simulink model "ITSC2021_CoupledPathFollowingSim_discrete"  (R2019b)
settings: Solver=FixedStepAuto  StartTime=0.0  StopTime=50  FixedStep=0.01  RelTol=1e-4  EnableMultiTasking=on
values from neighbouring files (symbols this model uses):
  friction_grid_cluster = [frictionGrid_Cluster_table.position_x, frictionGrid_Cluster_table.position_y, frictionGrid_Cluster_table.position_z, frictionGrid_Cluster_table.friction_coefficient]    [ITSC2021_runCoupledPathFollowingSim.m]
  inputTrajectory = inputTrajectory(unique_station_indices,:)    [ITSC2021_runCoupledPathFollowingSim.m]
  road_geometry = [sectionRef_table.east, sectionRef_table.north, sectionRef_table.up, sectionRef_table.grade, sectionRef_table.bank, road_geometry_radius, sectionRef_table.yaw]    [ITSC2021_runCoupledPathFollowingSim.m]
undefined symbols (not defined in the file or in its folder): DiscIntNeverNeededParam, flag, initial, mdlparam, mdlParam
libraries: simulink x6, autolibshared x1
(part 2 of 3)

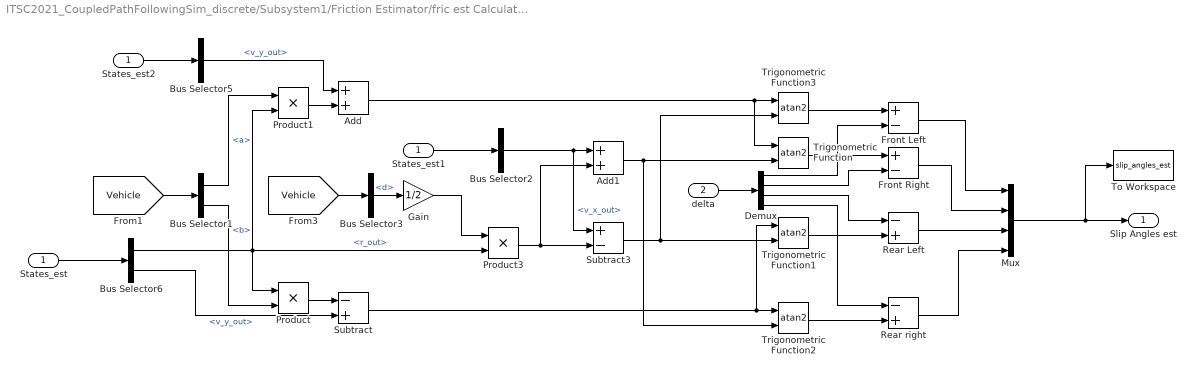
== system ITSC2021_CoupledPathFollowingSim_discrete/Subsystem1/Friction Estimator/fric est Calculate Slips ==
  States_est : Inport
  delta : Inport  Port=2
  Add : Sum
  Add1 : Sum
  Bus Selector1 : BusSelector  OutputSignals=a,b
  Bus Selector2 : BusSelector  OutputSignals=v_x_out
  Bus Selector3 : BusSelector  OutputSignals=d
  Bus Selector5 : BusSelector  OutputSignals=v_y_out
  Bus Selector6 : BusSelector  OutputSignals=r_out,v_y_out
  Demux : Demux
  Front Left : Sum  Inputs=+-
  Front Right : Sum  Inputs=+-
  Gain : Gain  Gain=1/2
  Mux : Mux
  Product : Product  RndMeth=Zero
  Product1 : Product  RndMeth=Zero
  Product3 : Product  RndMeth=Zero
  Rear Left : Sum  Inputs=-+
  Rear right : Sum  Inputs=-+
  States_est1 : InportShadow
  States_est2 : InportShadow
  Subtract : Sum  Inputs=-+
  Subtract3 : Sum  Inputs=+-
  To Workspace : ToWorkspace  VariableName=slip_angles_est  SampleTime=-1
  Trigonometric Function{,1..3} (4 alike) : Trigonometry  Operator=atan2
  Slip Angles est : Outport
  wires:
  Product1/1 -> Add/2
  Trigonometric Function3/1 -> Front Left/1
  Bus Selector1/1 -> Product1/1  "<a>"
  [Vehicle] -> Bus Selector3/1
  Front Left/1 -> Mux/1
  Front Right/1 -> Mux/2
  Bus Selector1/2 -> Product/2  "<b>"
  Trigonometric Function2/1 -> Rear right/2
  Mux/1 -> Slip Angles est/1, To Workspace/1
  Product/1 -> Subtract/1
  [Vehicle] -> Bus Selector1/1
  Add/1 -> Trigonometric Function3/1, Trigonometric Function/1
  Demux/3 -> Rear Left/1
  Demux/4 -> Rear right/1
  Bus Selector3/1 -> Gain/1  "<d>"
  Rear right/1 -> Mux/4
  Rear Left/1 -> Mux/3
  delta/1 -> Demux/1
  Gain/1 -> Product3/1
  Trigonometric Function/1 -> Front Right/1
  Subtract3/1 -> Trigonometric Function1/2, Trigonometric Function3/2
  Trigonometric Function1/1 -> Rear Left/2
  States_est/1 -> Bus Selector6/1
  Demux/2 -> Front Right/2
  Bus Selector6/2 -> Subtract/2  "<v_y_out>"
  Product3/1 -> Subtract3/2, Add1/2
  Add1/1 -> Trigonometric Function/2, Trigonometric Function2/2
  Subtract/1 -> Trigonometric Function2/1, Trigonometric Function1/1
  Demux/1 -> Front Left/2
  Bus Selector6/1 -> Product/1, Product1/2, Product3/2  "<r_out>"
  Bus Selector2/1 -> Subtract3/1, Add1/1  "<v_x_out>"
  States_est1/1 -> Bus Selector2/1
  States_est2/1 -> Bus Selector5/1
  Bus Selector5/1 -> Add/1  "<v_y_out>"

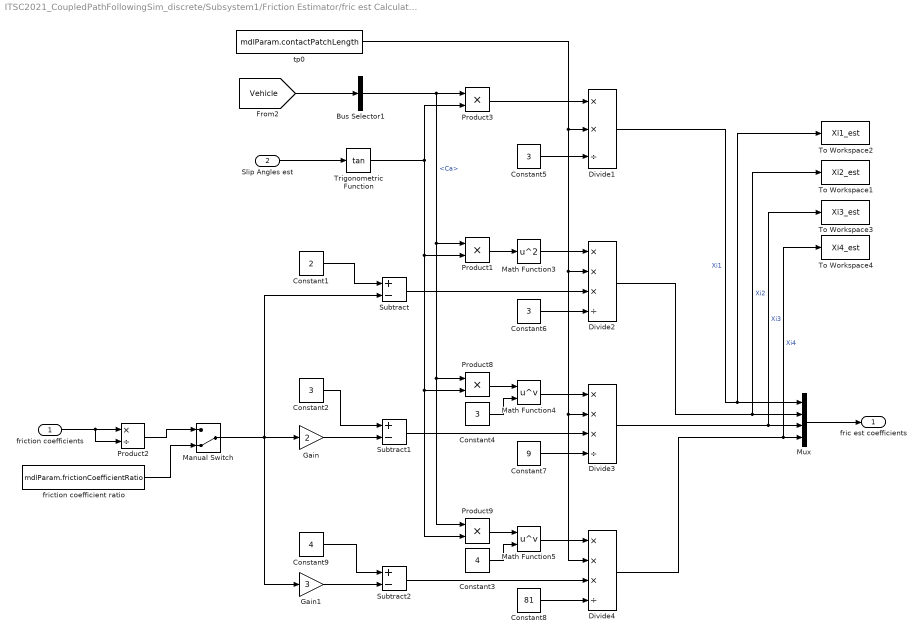
== system ITSC2021_CoupledPathFollowingSim_discrete/Subsystem1/Friction Estimator/fric est Calculate Xis ==
  friction coefficients : Inport
  Slip Angles est : Inport  Port=2
  Bus Selector1 : BusSelector  OutputSignals=Ca
  Constant1 : Constant  Value=2
  Constant{2,4..6} (4 alike) : Constant  Value=3
  Constant3 : Constant  Value=4
  Constant7 : Constant  Value=9
  Constant8 : Constant  Value=81
  Constant9 : Constant  Value=4
  Divide1 : Product  Inputs=**/
  Divide2 : Product  Inputs=***/
  Divide3 : Product  Inputs=***/
  Divide4 : Product  Inputs=***/
  Gain : Gain  Gain=2
  Gain1 : Gain  Gain=3
  Manual Switch : ManualSwitch  CurrentSetting=0
  Math Function3 : Math  Operator=square  SaturateOnIntegerOverflow=on
  Math Function4 : Math  Operator=pow  SignedPower=off  SaturateOnIntegerOverflow=on
  Math Function5 : Math  Operator=pow  SignedPower=off  SaturateOnIntegerOverflow=on
  Mux : Mux
  Product{1,3,8..9} (4 alike) : Product  RndMeth=Zero
  Product2 : Product  Inputs=*/  RndMeth=Zero
  Subtract : Sum  Inputs=+-
  Subtract1 : Sum  Inputs=+-
  Subtract2 : Sum  Inputs=+-
  To Workspace1 : ToWorkspace  VariableName=Xi2_est  SampleTime=-1
  To Workspace2 : ToWorkspace  VariableName=Xi1_est  SampleTime=-1
  To Workspace3 : ToWorkspace  VariableName=Xi3_est  SampleTime=-1
  To Workspace4 : ToWorkspace  VariableName=Xi4_est  SampleTime=-1
  Trigonometric Function : Trigonometry  Operator=tan
  friction coefficient ratio : Constant  Value=mdlParam.frictionCoefficientRatio
  tp0 : Constant  Value=mdlParam.contactPatchLength
  fric est coefficients : Outport
  wires:
  Mux/1 -> fric est coefficients/1
  Trigonometric Function/1 -> Product1/2, Product8/2, Product9/2, Product3/2
  tp0/1 -> Divide4/2, Divide3/2, Divide2/2, Divide1/2
  Bus Selector1/1 -> Product9/1, Product8/1, Product1/1, Product3/1  "<Ca>"
  Constant3/1 -> Math Function5/2
  Constant4/1 -> Math Function4/2
  Math Function3/1 -> Divide2/1
  Product1/1 -> Math Function3/1
  [Vehicle] -> Bus Selector1/1
  Math Function4/1 -> Divide3/1
  Constant5/1 -> Divide1/3
  Slip Angles est/1 -> Trigonometric Function/1
  Math Function5/1 -> Divide4/1
  Product8/1 -> Math Function4/1
  Product9/1 -> Math Function5/1
  Constant7/1 -> Divide3/4
  Product3/1 -> Divide1/1
  Subtract1/1 -> Divide3/3
  Constant1/1 -> Subtract/1
  Constant2/1 -> Subtract1/1
  Manual Switch/1 -> Gain1/1, Subtract/2, Gain/1
  Gain/1 -> Subtract1/2
  Constant9/1 -> Subtract2/1
  Gain1/1 -> Subtract2/2
  Constant6/1 -> Divide2/4
  Subtract/1 -> Divide2/3
  Constant8/1 -> Divide4/4
  Subtract2/1 -> Divide4/3
  Divide1/1 -> To Workspace2/1, Mux/1  "Xi1"
  Divide4/1 -> To Workspace4/1, Mux/4  "Xi4"
  Divide2/1 -> To Workspace1/1, Mux/2  "Xi2"
  Divide3/1 -> To Workspace3/1, Mux/3  "Xi3"
  friction coefficients/1 -> Product2/2, Product2/1
  Product2/1 -> Manual Switch/1
  friction coefficient ratio/1 -> Manual Switch/2

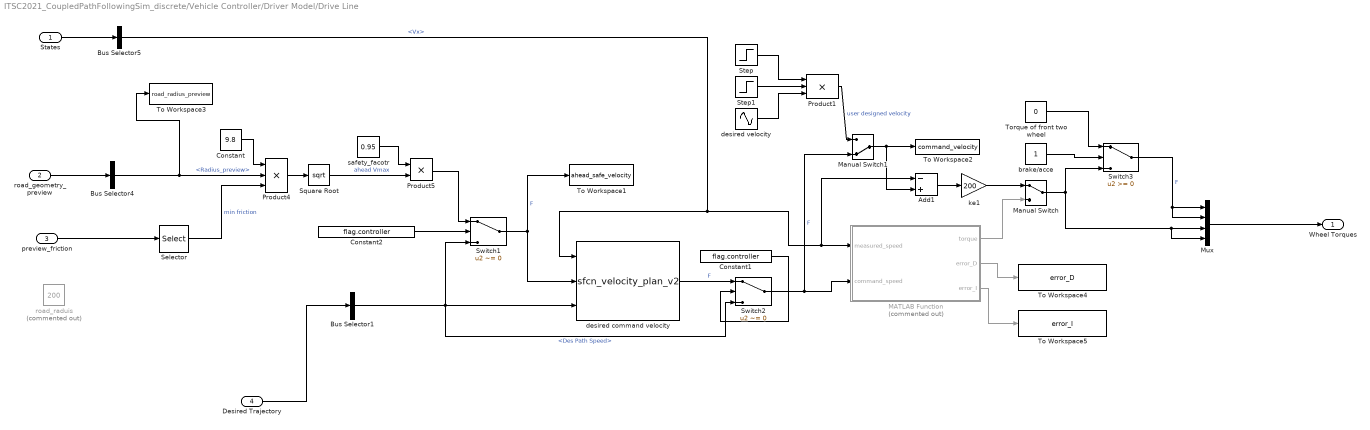
== system ITSC2021_CoupledPathFollowingSim_discrete/Vehicle Controller/Driver Model/Drive Line ==
  States : Inport
  road_geometry_preview : Inport  Port=2
  preview_friction : Inport  Port=3
  Desired Trajectory : Inport  Port=4
  Add1 : Sum  Inputs=-+
  Bus Selector1 : BusSelector  OutputSignals=Des Path Speed
  Bus Selector4 : BusSelector  OutputSignals=Radius_preview
  Bus Selector5 : BusSelector  OutputSignals=Vx
  Constant : Constant  Value=9.8
  Constant1 : Constant  Value=flag.controller
  Constant2 : Constant  Value=flag.controller
  MATLAB Function : MATLAB Function  Commented=on  TreatAsAtomicUnit=on
  Manual Switch : ManualSwitch
      settings: AttributesFormatString=%<BlockType>
  Manual Switch1 : ManualSwitch  CurrentSetting=0
  Mux : Mux
  Product1 : Product  Inputs=3  SaturateOnIntegerOverflow=on  OutDataTypeStr=Inherit: Same as first input
  Product4 : Product  Inputs=3
  Product5 : Product
  Selector : Selector  InputPortWidth=5  IndexOptions=Index vector (dialog)  Indices=[3]  OutputSizes=1
  Square Root : Sqrt  SaturateOnIntegerOverflow=on
  Step : Step  Time=2  Before=1  After=0.8  SampleTime=0.01
  Step1 : Step  Time=20  Before=1  After=1.2  SampleTime=0.01
  Switch1 : Switch  Criteria=u2 ~= 0  ZeroCross=off
  Switch2 : Switch  Criteria=u2 ~= 0  ZeroCross=off
  Switch3 : Switch  ZeroCross=off
  To Workspace1 : ToWorkspace  VariableName=ahead_safe_velocity  SampleTime=-1
      settings: Save2DSignal=2-D array (concatenate along first dimension)
  To Workspace2 : ToWorkspace  VariableName=command_velocity  SampleTime=-1
      settings: Save2DSignal=2-D array (concatenate along first dimension)
  To Workspace3 : ToWorkspace  VariableName=road_radius_preview  SampleTime=-1
      settings: Save2DSignal=2-D array (concatenate along first dimension)
  To Workspace4 : ToWorkspace  VariableName=error_D  SampleTime=-1
      settings: Save2DSignal=2-D array (concatenate along first dimension)
  To Workspace5 : ToWorkspace  VariableName=error_I  SampleTime=-1
      settings: Save2DSignal=2-D array (concatenate along first dimension)
  Torque of front two wheel : Constant  Value=0
  brake/acce : Constant
  desired command velocity : M-S-Function  FunctionName=sfcn_velocity_plan_v2
  desired velocity : Sin  SineType=Sample based  Amplitude=0  Bias=27.392001251200000  Frequency=0.1*2*pi  Samples=2000  SampleTime=0.01
  ke1 : Gain  Gain=200
  road_raduis : Constant  Commented=on  Value=200
  safety_facotr : Constant  Value=0.95
  Wheel Torques : Outport
  wires:
  Product4/1 -> Square Root/1
  Add1/1 -> ke1/1
  States/1 -> Bus Selector5/1
  Switch2/1 -> Manual Switch1/2, MATLAB Function/2(command_speed)  "F"
  Bus Selector5/1 -> Add1/1, MATLAB Function/1(measured_speed), desired command velocity/1  "<Vx>"
  Switch3/1 -> Mux/2, Mux/1  "F"
  Bus Selector1/1 -> Switch1/3, Switch2/3, desired command velocity/3  "<Des Path Speed>"
  Torque of front two wheel/1 -> Switch3/1
  Product5/1 -> Switch1/1
  Selector/1 -> Product4/3  "min friction"
  MATLAB Function/3(error_I) -> To Workspace5/1
  MATLAB Function/2(error_D) -> To Workspace4/1
  Manual Switch/1 -> Mux/4, Mux/3, Switch3/3
  Bus Selector4/1 -> To Workspace3/1, Product4/2  "<Radius_preview>"
  desired command velocity/1 -> Switch2/1  "F"
  Constant/1 -> Product4/1
  Constant2/1 -> Switch1/2
  Square Root/1 -> Product5/2  "ahead Vmax"
  brake/acce/1 -> Switch3/2
  Desired Trajectory/1 -> Bus Selector1/1
  Switch1/1 -> desired command velocity/2, To Workspace1/1  "F"
  ke1/1 -> Manual Switch/1
  safety_facotr/1 -> Product5/1
  MATLAB Function/1(torque) -> Manual Switch/2
  Constant1/1 -> Switch2/2
  road_geometry_preview/1 -> Bus Selector4/1
  preview_friction/1 -> Selector/1
  Mux/1 -> Wheel Torques/1
  desired velocity/1 -> Product1/3
  Step/1 -> Product1/1
  Product1/1 -> Manual Switch1/1  "user designed velocity"
  Step1/1 -> Product1/2
  Manual Switch1/1 -> To Workspace2/1, Add1/2

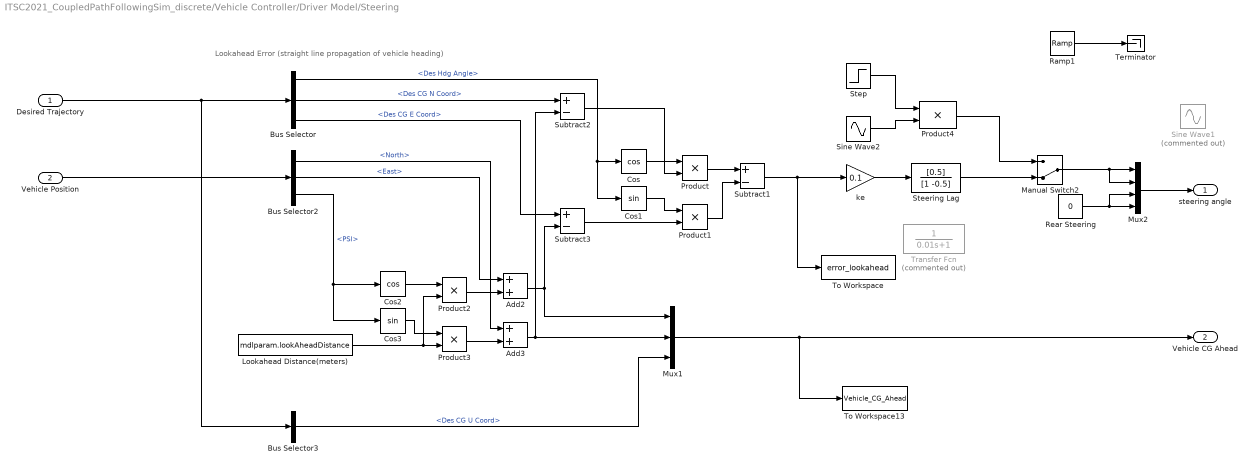
== system ITSC2021_CoupledPathFollowingSim_discrete/Vehicle Controller/Driver Model/Steering ==
  note: Lookahead Error (straight line propagation of vehicle heading)
  Desired Trajectory : Inport
  Vehicle Position : Inport  Port=2
  Add2 : Sum
  Add3 : Sum
  Bus Selector : BusSelector  OutputSignals=Des Hdg Angle,Des CG N Coord,Des CG E Coord
  Bus Selector2 : BusSelector  OutputSignals=North,East,PSI
  Bus Selector3 : BusSelector  OutputSignals=Des CG U Coord
  Cos : Trigonometry  Operator=cos
  Cos1 : Trigonometry
  Cos2 : Trigonometry  Operator=cos
  Cos3 : Trigonometry
  Lookahead Distance(meters) : Constant  Value=mdlparam.lookAheadDistance
  Manual Switch2 : ManualSwitch  CurrentSetting=0
  Mux1 : Mux  Inputs=3
  Mux2 : Mux
  Product{,1..3} (4 alike) : Product
  Product4 : Product  SaturateOnIntegerOverflow=on  OutDataTypeStr=Inherit: Same as first input
  Ramp1 : simulink/Sources/Ramp  slope=0.1  start=0  InitialOutput=0
  Rear Steering : Constant  Value=0
  Sine Wave1 : Sin  Commented=on  SampleTime=0
  Sine Wave2 : Sin  SineType=Sample based  Amplitude=0*pi/180  Frequency=0.1*2*pi  Samples=2000  SampleTime=0.01
  Steering Lag : DiscreteFilter  Numerator=[0.5]  Denominator=[1 -0.5]
  Step : Step  Time=40  Before=1  After=0  SampleTime=0.01
  Subtract1 : Sum  Inputs=+-
  Subtract2 : Sum  Inputs=+-
  Subtract3 : Sum  Inputs=+-
  Terminator : Terminator
  To Workspace : ToWorkspace  VariableName=error_lookahead  SampleTime=-1
      settings: Save2DSignal=2-D array (concatenate along first dimension)
  To Workspace13 : ToWorkspace  VariableName=Vehicle_CG_Ahead  SampleTime=-1
      settings: Save2DSignal=2-D array (concatenate along first dimension)
  Transfer Fcn : TransferFcn  Commented=on  Denominator=[0.01 1]
  ke : Gain  Gain=0.1
  steering angle : Outport
  Vehicle CG Ahead : Outport  Port=2
  wires:
  ke/1 -> Steering Lag/1
  Subtract2/1 -> Product/2
  Mux2/1 -> steering angle/1
  Lookahead Distance(meters)/1 -> Product2/2, Product3/2
  Bus Selector/3 -> Subtract3/1  "<Des CG E Coord>"
  Subtract3/1 -> Product1/2
  Cos1/1 -> Product1/1
  Add3/1 -> Subtract2/2, Mux1/2
  Bus Selector2/2 -> Add2/1  "<East>"
  Add2/1 -> Mux1/1, Subtract3/2
  Bus Selector2/1 -> Add3/1  "<North>"
  Cos3/1 -> Product3/1
  Rear Steering/1 -> Mux2/3, Mux2/4
  Desired Trajectory/1 -> Bus Selector3/1, Bus Selector/1
  Product/1 -> Subtract1/1
  Ramp1/1 -> Terminator/1
  Mux1/1 -> Vehicle CG Ahead/1, To Workspace13/1
  Bus Selector2/3 -> Cos3/1, Cos2/1  "<PSI>"
  Vehicle Position/1 -> Bus Selector2/1
  Bus Selector3/1 -> Mux1/3  "<Des CG U Coord>"
  Cos2/1 -> Product2/1
  Product3/1 -> Add3/2
  Subtract1/1 -> To Workspace/1, ke/1
  Product2/1 -> Add2/2
  Product1/1 -> Subtract1/2
  Bus Selector/2 -> Subtract2/1  "<Des CG N Coord>"
  Bus Selector/1 -> Cos/1, Cos1/1  "<Des Hdg Angle>"
  Cos/1 -> Product/1
  Step/1 -> Product4/1
  Sine Wave2/1 -> Product4/2
  Manual Switch2/1 -> Mux2/2, Mux2/1
  Product4/1 -> Manual Switch2/1
  Steering Lag/1 -> Manual Switch2/2

== system ITSC2021_CoupledPathFollowingSim_discrete/Vehicle Dynamics/Calculate Normals/Normal Force Lateral Transfer ==
  Accelerations : Inport
  Bus Selector1 : BusSelector  OutputSignals=ay
  Bus Selector4 : BusSelector  OutputSignals=b,L,a
  Bus Selector6 : BusSelector  OutputSignals=m,h_cg,d
  Delay1 : Delay  DelayLength=1  InitialCondition=0
  Divide3 : Product  Inputs=*/
  Divide4 : Product  Inputs=/*
  Gain2 : Gain  Gain=0
  Product{1..2,4..5} (4 alike) : Product  RndMeth=Zero
  Product3 : Product  Inputs=*/  RndMeth=Zero
  Lateral Transfer Front : Outport
  Lateral Transfer Rear : Outport  Port=2
  wires:
  Divide3/1 -> Product2/2
  Bus Selector4/2 -> Divide3/2, Divide4/1  "<L>"
  Bus Selector4/1 -> Divide3/1  "<b>"
  Gain2/1 -> Product5/1
  Product2/1 -> Lateral Transfer Front/1
  Product5/1 -> Product2/1, Product1/2
  Bus Selector6/2 -> Product3/1  "<h_cg>"
  Product1/1 -> Lateral Transfer Rear/1
  Bus Selector6/1 -> Product4/2  "<m>"
  Accelerations/1 -> Delay1/1
  Delay1/1 -> Bus Selector1/1
  Divide4/1 -> Product1/1
  Bus Selector1/1 -> Product4/1  "<ay>"
  Bus Selector6/3 -> Product3/2  "<d>"
  [Vehicle] -> Bus Selector4/1
  [Vehicle] -> Bus Selector6/1
  Bus Selector4/3 -> Divide4/2  "<a>"
  Product4/1 -> Gain2/1
  Product3/1 -> Product5/2

== system ITSC2021_CoupledPathFollowingSim_discrete/Vehicle Dynamics/Calculate Normals/Normal Force Longitudinal Transfer ==
  Accelerations : Inport
  Bus Selector2 : BusSelector  OutputSignals=m,L,h_cg
  Bus Selector3 : BusSelector  OutputSignals=ax
  Delay : Delay  DelayLength=1  InitialCondition=0
  Divide1 : Product  Inputs=/*
  Gain1 : Gain  Gain=0
  Gain3 : Gain  Gain=2
  Product1 : Product  RndMeth=Zero
  Product2 : Product  RndMeth=Zero
  Half Long Transfer : Outport
  wires:
  Bus Selector2/2 -> Gain3/1  "<L>"
  Gain1/1 -> Product1/1
  Bus Selector2/3 -> Divide1/2  "<h_cg>"
  Divide1/1 -> Product1/2
  [Vehicle] -> Bus Selector2/1
  Accelerations/1 -> Delay/1
  Bus Selector2/1 -> Product2/2  "<m>"
  Bus Selector3/1 -> Product2/1  "<ax>"
  Product2/1 -> Gain1/1
  Product1/1 -> Half Long Transfer/1
  Gain3/1 -> Divide1/1
  Delay/1 -> Bus Selector3/1

== system ITSC2021_CoupledPathFollowingSim_discrete/Vehicle Dynamics/Calculate Normals/Normal Force Static ==
  Road Geometry : Inport
  " " : Product  RndMeth=Zero
  Add : Sum
  Bus Selector : BusSelector  OutputSignals=Grade
  Bus Selector1 : BusSelector  OutputSignals=m,L,h_cg,b,a
  Divide : Product  Inputs=*/
  Gain : Gain  Gain=2
  Mux1 : Mux
  Product1 : Product  RndMeth=Zero
  Product3 : Product  Inputs=3  RndMeth=Zero
  Product4 : Product  RndMeth=Zero
  Subtract : Sum  Inputs=-+
  To Workspace4 : ToWorkspace  VariableName=FzStatic  SampleTime=-1
  Trigonometric Function : Trigonometry  Operator=cos
  Trigonometric Function1 : Trigonometry  Operator=tan
  g : Constant  Value=9.81
  Half Static Front : Outport
  Half Static Rear : Outport  Port=2
  wires:
  Product4/1 -> Add/1, Subtract/1
  Add/1 -> Product1/2
  g/1 -> Product3/2
  [Vehicle] -> Bus Selector1/1
  Bus Selector1/4 -> Subtract/2  "<b>"
  Product3/1 -> Divide/1
  Bus Selector1/1 -> Product3/3  "<m>"
  Trigonometric Function/1 -> Product3/1
  Bus Selector1/5 -> Add/2  "<a>"
  Bus Selector1/3 -> Product4/2  "<h_cg>"
  Trigonometric Function1/1 -> Product4/1
  Divide/1 -> Product1/1, " "/1
  Bus Selector/1 -> Trigonometric Function1/1, Trigonometric Function/1  "<Grade>"
  Bus Selector1/2 -> Gain/1  "<L>"
  Subtract/1 -> " "/2
  Gain/1 -> Divide/2
  Road Geometry/1 -> Bus Selector/1
  Product1/1 -> Mux1/4, Mux1/3, Half Static Rear/1
  Mux1/1 -> To Workspace4/1
  " "/1 -> Half Static Front/1, Mux1/1, Mux1/2

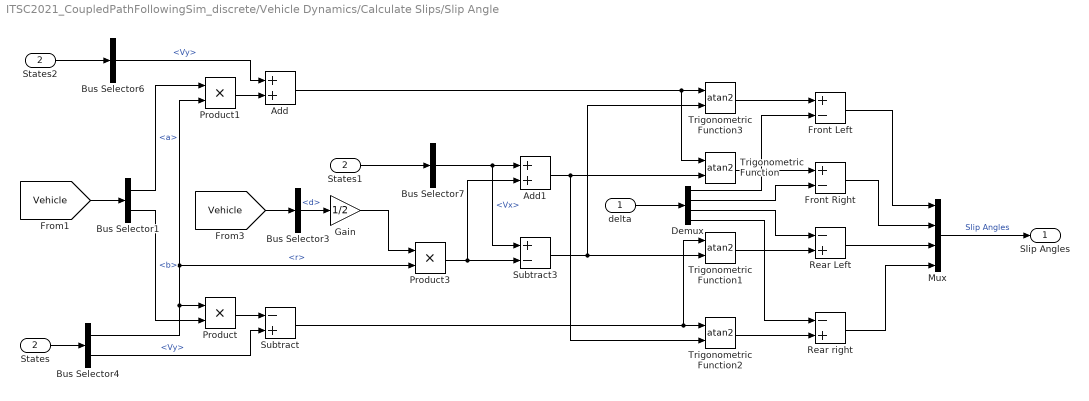
== system ITSC2021_CoupledPathFollowingSim_discrete/Vehicle Dynamics/Calculate Slips/Slip Angle ==
  delta : Inport
  States : Inport  Port=2
  Add : Sum
  Add1 : Sum
  Bus Selector1 : BusSelector  OutputSignals=a,b
  Bus Selector3 : BusSelector  OutputSignals=d
  Bus Selector4 : BusSelector  OutputSignals=r,Vy
  Bus Selector6 : BusSelector  OutputSignals=Vy
  Bus Selector7 : BusSelector  OutputSignals=Vx
  Demux : Demux
  Front Left : Sum  Inputs=+-
  Front Right : Sum  Inputs=+-
  Gain : Gain  Gain=1/2
  Mux : Mux
  Product : Product  RndMeth=Zero
  Product1 : Product  RndMeth=Zero
  Product3 : Product  RndMeth=Zero
  Rear Left : Sum  Inputs=-+
  Rear right : Sum  Inputs=-+
  States1 : InportShadow  Port=2
  States2 : InportShadow  Port=2
  Subtract : Sum  Inputs=-+
  Subtract3 : Sum  Inputs=+-
  Trigonometric Function{,1..3} (4 alike) : Trigonometry  Operator=atan2
  Slip Angles : Outport
  wires:
  States1/1 -> Bus Selector7/1
  Bus Selector4/1 -> Product1/2, Product3/2, Product/1  "<r>"
  Demux/1 -> Front Left/2
  Subtract/1 -> Trigonometric Function2/1, Trigonometric Function1/1
  Add1/1 -> Trigonometric Function/2, Trigonometric Function2/2
  Product3/1 -> Subtract3/2, Add1/2
  Demux/2 -> Front Right/2
  Trigonometric Function1/1 -> Rear Left/2
  Subtract3/1 -> Trigonometric Function1/2, Trigonometric Function3/2
  Trigonometric Function/1 -> Front Right/1
  Gain/1 -> Product3/1
  delta/1 -> Demux/1
  Rear Left/1 -> Mux/3
  Rear right/1 -> Mux/4
  Bus Selector3/1 -> Gain/1  "<d>"
  Demux/4 -> Rear right/1
  Demux/3 -> Rear Left/1
  Add/1 -> Trigonometric Function/1, Trigonometric Function3/1
  [Vehicle] -> Bus Selector1/1
  Product/1 -> Subtract/1
  Mux/1 -> Slip Angles/1  "Slip Angles"
  Trigonometric Function2/1 -> Rear right/2
  Bus Selector1/2 -> Product/2  "<b>"
  Front Right/1 -> Mux/2
  Front Left/1 -> Mux/1
  [Vehicle] -> Bus Selector3/1
  Bus Selector1/1 -> Product1/1  "<a>"
  Trigonometric Function3/1 -> Front Left/1
  Product1/1 -> Add/2
  Bus Selector7/1 -> Subtract3/1, Add1/1  "<Vx>"
  States2/1 -> Bus Selector6/1
  Bus Selector4/2 -> Subtract/2  "<Vy>"
  Bus Selector6/1 -> Add/1  "<Vy>"
  States/1 -> Bus Selector4/1

== system ITSC2021_CoupledPathFollowingSim_discrete/Vehicle Dynamics/Calculate Slips/Wheel Slip Ratio this block is wrong because it use vehicle body velocity to calculate slip ratio ==
  note: κ>0, acceleration→ positive Fx
      | κ<0, braking → negative Fx
  States : Inport
  Anti-Divide by Zero : Subsystem
  Bus Selector2 : BusSelector  OutputSignals=Re
  Bus Selector4 : BusSelector  OutputSignals=Vx,omega
  Divide2 : Product  Inputs=/*
  Product2 : Product  RndMeth=Zero
  Saturation : Saturate  UpperLimit=1  LowerLimit=-1  ZeroCross=off
  Subtract2 : Sum  Inputs=-+
  Switch1 : Switch  Criteria=u2 > Threshold  ZeroCross=off  SaturateOnIntegerOverflow=on
  zero Wheel Slip : Constant  Value=[0 0 0 0]
  Wheel Slips : Outport
  wires:
  Subtract2/1 -> Divide2/2
  Anti-Divide by Zero/1(Out1) -> Divide2/1
  zero Wheel Slip/1 -> Switch1/3
  Bus Selector4/1 -> Anti-Divide by Zero/1(In1), Subtract2/1, Switch1/2  "<Vx>"
  Bus Selector2/1 -> Product2/1  "<Re>"
  [Vehicle] -> Bus Selector2/1
  Divide2/1 -> Switch1/1
  Switch1/1 -> Saturation/1
  Product2/1 -> Subtract2/2
  Saturation/1 -> Wheel Slips/1  "Wheel Slips"
  Bus Selector4/2 -> Product2/2  "<omega>"
  States/1 -> Bus Selector4/1

== system ITSC2021_CoupledPathFollowingSim_discrete/Vehicle Dynamics/Calculate Slips/Wheel Slip Ratio1 ==
  note: κ>0, acceleration→ positive Fx
      | κ<0, braking → negative Fx
  Vtire,x : Inport
  States : Inport  Port=2
  Anti-Divide by Zero : Subsystem
  Bus Selector2 : BusSelector  OutputSignals=Re
  Bus Selector4 : BusSelector  OutputSignals=omega
  Divide2 : Product  Inputs=/*
  Max : MinMax  Function=max  Inputs=2
  Product2 : Product  RndMeth=Zero
  Saturation : Saturate  UpperLimit=0.9  LowerLimit=-0.9  ZeroCross=off
  Subtract2 : Sum  Inputs=-+
  Switch1 : Switch  Criteria=u2 > Threshold  ZeroCross=off  SaturateOnIntegerOverflow=on
  Terminator2 : Terminator
  zero Wheel Slip : Constant  Value=[0 0 0 0]
  Wheel Slips Ratio : Outport
  wires:
  Subtract2/1 -> Divide2/2
  Anti-Divide by Zero/1(Out1) -> Divide2/1
  zero Wheel Slip/1 -> Switch1/3
  Vtire,x/1 -> Max/1, Anti-Divide by Zero/1(In1), Subtract2/1, Switch1/2
  Bus Selector2/1 -> Product2/2  "<Re>"
  [Vehicle] -> Bus Selector2/1
  Divide2/1 -> Switch1/1
  Switch1/1 -> Saturation/1
  Product2/1 -> Max/2, Subtract2/2
  Saturation/1 -> Wheel Slips Ratio/1  "Wheel Slips"
  Bus Selector4/1 -> Product2/1  "<omega>"
  States/1 -> Bus Selector4/1
  Max/1 -> Terminator2/1

== system ITSC2021_CoupledPathFollowingSim_discrete/Vehicle Dynamics/Calculate Slips/vehicle2tire ==
  States : Inport
  delta : Inport  Port=2
  Add : Sum
  Add1 : Sum
  Add2 : Sum
  Add3 : Sum  Inputs=-+
  Bus Selector1 : BusSelector  OutputSignals=d,a,b
  Bus Selector4 : BusSelector  OutputSignals=r,Vy
  Bus Selector7 : BusSelector  OutputSignals=Vx
  Cos : Trigonometry  Operator=cos
  Gain : Gain  Gain=1/2
  Mux1 : Mux
  Mux2 : Mux
  Product{,1..6} (7 alike) : Product  RndMeth=Zero
  Sin : Trigonometry
  States2 : InportShadow
  Subtract : Sum  Inputs=-+
  Subtract3 : Sum  Inputs=+-
  To Workspace1 : ToWorkspace  VariableName=Vaxle_y  SampleTime=-1
      settings: Save2DSignal=2-D array (concatenate along first dimension)
  To Workspace4 : ToWorkspace  VariableName=Vaxle_x  SampleTime=-1
      settings: Save2DSignal=2-D array (concatenate along first dimension)
  Vtire,x : Outport
  Vtire,y : Outport  Port=2
  wires:
  States2/1 -> Bus Selector7/1
  Bus Selector4/1 -> Product3/2, Product1/2, Product/1  "<r>"
  Bus Selector1/2 -> Product1/1  "<a>"
  Product3/1 -> Subtract3/2, Add1/2
  Bus Selector7/1 -> Add1/1, Subtract3/1  "<Vx>"
  Product/1 -> Subtract/1
  Bus Selector4/2 -> Add/2, Subtract/2  "<Vy>"
  [Vehicle] -> Bus Selector1/1
  Product1/1 -> Add/1
  Add/1 -> Mux1/1, Mux1/2  "Vy+ar"
  Mux2/1 -> Product2/1, Product5/1, To Workspace4/1  "Vaxle_x"
  Mux1/1 -> Product4/2, Product6/2, To Workspace1/1  "Vaxle_y"
  Bus Selector1/3 -> Product/2  "<b>"
  Gain/1 -> Product3/1
  States/1 -> Bus Selector4/1
  Subtract/1 -> Mux1/4, Mux1/3  "Vy-br"
  Bus Selector1/1 -> Gain/1  "<d>"
  Subtract3/1 -> Mux2/1, Mux2/3  "Vx-rd/2"
  Add1/1 -> Mux2/4, Mux2/2  "Vx+rd/2"
  Product2/1 -> Add2/1
  Add2/1 -> Vtire,x/1
  Add3/1 -> Vtire,y/1
  delta/1 -> Sin/1, Cos/1
  Cos/1 -> Product6/1, Product2/2
  Sin/1 -> Product5/2, Product4/1
  Product4/1 -> Add2/2
  Product5/1 -> Add3/1
  Product6/1 -> Add3/2

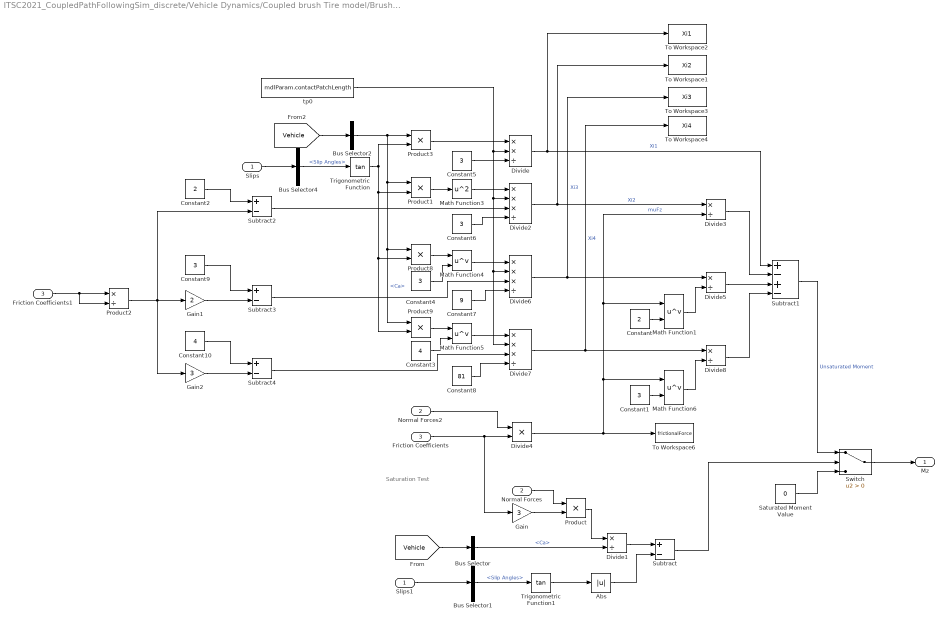
== system ITSC2021_CoupledPathFollowingSim_discrete/Vehicle Dynamics/Coupled brush Tire model/Brush Aligning Moment Model ==
  note: Saturation Test
  Slips : Inport
  Normal Forces : Inport  Port=2
  Friction Coefficients : Inport  Port=3
  Abs : Abs  ZeroCross=off
  Bus Selector : BusSelector  OutputSignals=Ca
  Bus Selector1 : BusSelector  OutputSignals=Slip Angles
  Bus Selector2 : BusSelector  OutputSignals=Ca
  Bus Selector4 : BusSelector  OutputSignals=Slip Angles
  Constant : Constant  Value=2
  Constant{1,4..6,9} (5 alike) : Constant  Value=3
  Constant10 : Constant  Value=4
  Constant2 : Constant  Value=2
  Constant3 : Constant  Value=4
  Constant7 : Constant  Value=9
  Constant8 : Constant  Value=81
  Divide : Product  Inputs=**/
  Divide{1,3,5,8} (4 alike) : Product  Inputs=*/
  Divide2 : Product  Inputs=***/
  Divide4 : Product
  Divide6 : Product  Inputs=***/
  Divide7 : Product  Inputs=***/
  Friction Coefficients1 : InportShadow  Port=3
  Gain : Gain  Gain=3
  Gain1 : Gain  Gain=2
  Gain2 : Gain  Gain=3
  Math Function{1,4..6} (4 alike) : Math  Operator=pow  SignedPower=off  SaturateOnIntegerOverflow=on
  Math Function3 : Math  Operator=square  SaturateOnIntegerOverflow=on
  Normal Forces2 : InportShadow  Port=2
  Product{,1,3,8..9} (5 alike) : Product  RndMeth=Zero
  Product2 : Product  Inputs=*/  RndMeth=Zero
  Saturated Moment Value : Constant  Value=0
  "Slips1 " : InportShadow
  Subtract{,2..4} (4 alike) : Sum  Inputs=+-
  Subtract1 : Sum  Inputs=+-+-
  Switch : Switch  Criteria=u2 > Threshold
  To Workspace1 : ToWorkspace  VariableName=Xi2  SampleTime=-1
  To Workspace2 : ToWorkspace  VariableName=Xi1  SampleTime=-1
  To Workspace3 : ToWorkspace  VariableName=Xi3  SampleTime=-1
  To Workspace4 : ToWorkspace  VariableName=Xi4  SampleTime=-1
  To Workspace6 : ToWorkspace  VariableName=frictionalForce  SampleTime=-1
  Trigonometric Function : Trigonometry  Operator=tan
  Trigonometric Function1 : Trigonometry  Operator=tan
  tp0 : Constant  Value=mdlParam.contactPatchLength
  Mz : Outport  VectorParamsAs1DForOutWhenUnconnected=off
  wires:
  Product/1 -> Divide1/1
  Switch/1 -> Mz/1
  Normal Forces2/1 -> Divide4/1
  Abs/1 -> Subtract/2
  Subtract/1 -> Switch/2
  Saturated Moment Value/1 -> Switch/3
  Bus Selector/1 -> Divide1/2  "<Ca>"
  [Vehicle] -> Bus Selector/1
  Divide1/1 -> Subtract/1
  Normal Forces/1 -> Product/1
  Gain/1 -> Product/2
  Trigonometric Function1/1 -> Abs/1
  Slips/1 -> Bus Selector4/1
  Subtract1/1 -> Switch/1  "Unsaturated Moment"
  "Slips1 "/1 -> Bus Selector1/1
  Divide4/1 -> Divide3/2, Math Function1/1, Math Function6/1, To Workspace6/1  "muFz"
  Constant/1 -> Math Function1/2
  [Vehicle] -> Bus Selector2/1
  Bus Selector2/1 -> Product9/1, Product8/1, Product1/1, Product3/1  "<Ca>"
  Constant3/1 -> Math Function5/2
  Constant4/1 -> Math Function4/2
  Trigonometric Function/1 -> Product1/2, Product9/2, Product8/2, Product3/2
  Product1/1 -> Math Function3/1
  Product8/1 -> Math Function4/1
  Product9/1 -> Math Function5/1
  tp0/1 -> Divide/2, Divide2/2, Divide7/2, Divide6/2
  Constant5/1 -> Divide/3
  Product3/1 -> Divide/1
  Math Function3/1 -> Divide2/1
  Constant7/1 -> Divide6/4
  Math Function4/1 -> Divide6/1
  Math Function5/1 -> Divide7/1
  Constant6/1 -> Divide2/4
  Constant8/1 -> Divide7/4
  Divide3/1 -> Subtract1/2
  Constant1/1 -> Math Function6/2
  Divide8/1 -> Subtract1/4
  Divide5/1 -> Subtract1/3
  Math Function6/1 -> Divide8/2
  Math Function1/1 -> Divide5/2
  Friction Coefficients/1 -> Divide4/2, Gain/1
  Divide/1 -> To Workspace2/1, Subtract1/1  "Xi1"
  Divide7/1 -> To Workspace4/1, Divide8/1  "Xi4"
  Divide2/1 -> To Workspace1/1, Divide3/1  "Xi2"
  Divide6/1 -> Divide5/1, To Workspace3/1  "Xi3"
  Gain2/1 -> Subtract4/2
  Product2/1 -> Gain2/1, Subtract2/2, Gain1/1
  Constant9/1 -> Subtract3/1
  Subtract3/1 -> Divide6/3
  Constant10/1 -> Subtract4/1
  Constant2/1 -> Subtract2/1
  Subtract2/1 -> Divide2/3
  Subtract4/1 -> Divide7/3
  Gain1/1 -> Subtract3/2
  Bus Selector4/1 -> Trigonometric Function/1  "<Slip Angles>"
  Bus Selector1/1 -> Trigonometric Function1/1  "<Slip Angles>"
  Friction Coefficients1/1 -> Product2/2, Product2/1

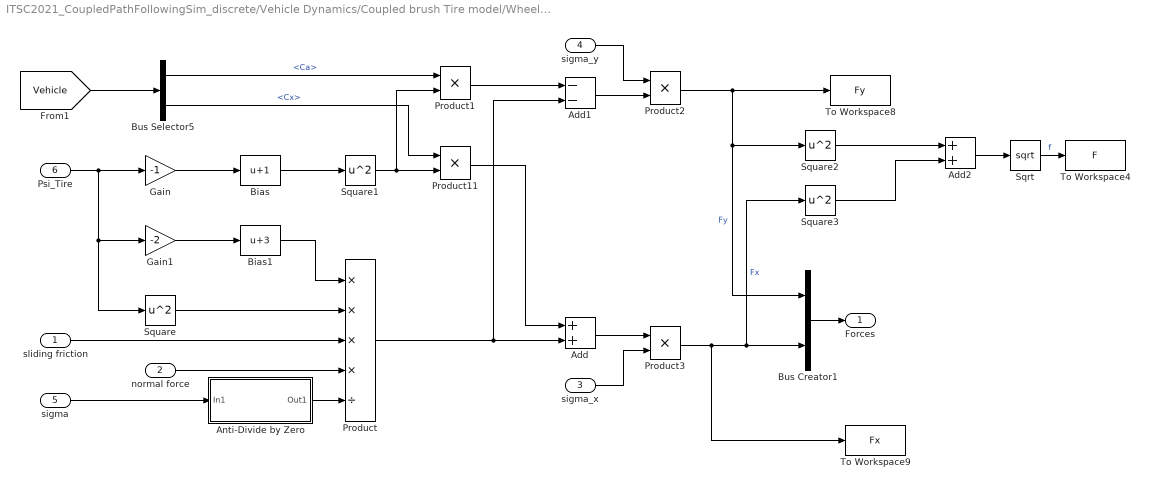
== system ITSC2021_CoupledPathFollowingSim_discrete/Vehicle Dynamics/Coupled brush Tire model/Wheel Forces ==
  sliding friction : Inport
  normal force : Inport  Port=2
  sigma_x : Inport  Port=3
  sigma_y : Inport  Port=4
  sigma : Inport  Port=5
  Psi_Tire : Inport  Port=6
  Add : Sum
  Add1 : Sum  Inputs=--
  Add2 : Sum
  Anti-Divide by Zero : Subsystem
  Bias : Bias  Bias=1
  Bias1 : Bias  Bias=3
  Bus Creator1 : BusCreator  Inputs=2
  Bus Selector5 : BusSelector  OutputSignals=Ca,Cx
  Gain : Gain  Gain=-1
  Gain1 : Gain  Gain=-2
  Product : Product  Inputs=****/
  Product{1..3,11} (4 alike) : Product  RndMeth=Zero
  Sqrt : Sqrt  SaturateOnIntegerOverflow=on
  Square{,1..3} (4 alike) : Math  Operator=square  SignedPower=off  SaturateOnIntegerOverflow=on
  To Workspace4 : ToWorkspace  VariableName=F  SampleTime=-1
  To Workspace8 : ToWorkspace  VariableName=Fy  SampleTime=-1
  To Workspace9 : ToWorkspace  VariableName=Fx  SampleTime=-1
  Forces : Outport
  wires:
  Product/1 -> Add1/2, Add/2
  Bus Selector5/2 -> Product11/1  "<Cx>"
  [Vehicle] -> Bus Selector5/1
  Gain/1 -> Bias/1
  Gain1/1 -> Bias1/1
  Bias/1 -> Square1/1
  Psi_Tire/1 -> Square/1, Gain1/1, Gain/1
  Square/1 -> Product/2
  Bias1/1 -> Product/1
  sliding friction/1 -> Product/3
  normal force/1 -> Product/4
  sigma/1 -> Anti-Divide by Zero/1(In1)
  Square1/1 -> Product1/2, Product11/2
  Product11/1 -> Add/1
  Bus Selector5/1 -> Product1/1  "<Ca>"
  Product1/1 -> Add1/1
  Add1/1 -> Product2/2
  sigma_y/1 -> Product2/1
  sigma_x/1 -> Product3/2
  Add/1 -> Product3/1
  Bus Creator1/1 -> Forces/1
  Product2/1 -> Bus Creator1/1, Square2/1, To Workspace8/1  "Fy"
  Product3/1 -> To Workspace9/1, Bus Creator1/2, Square3/1  "Fx"
  Square2/1 -> Add2/1
  Square3/1 -> Add2/2
  Add2/1 -> Sqrt/1
  Sqrt/1 -> To Workspace4/1  "f"
  Anti-Divide by Zero/1(Out1) -> Product/5

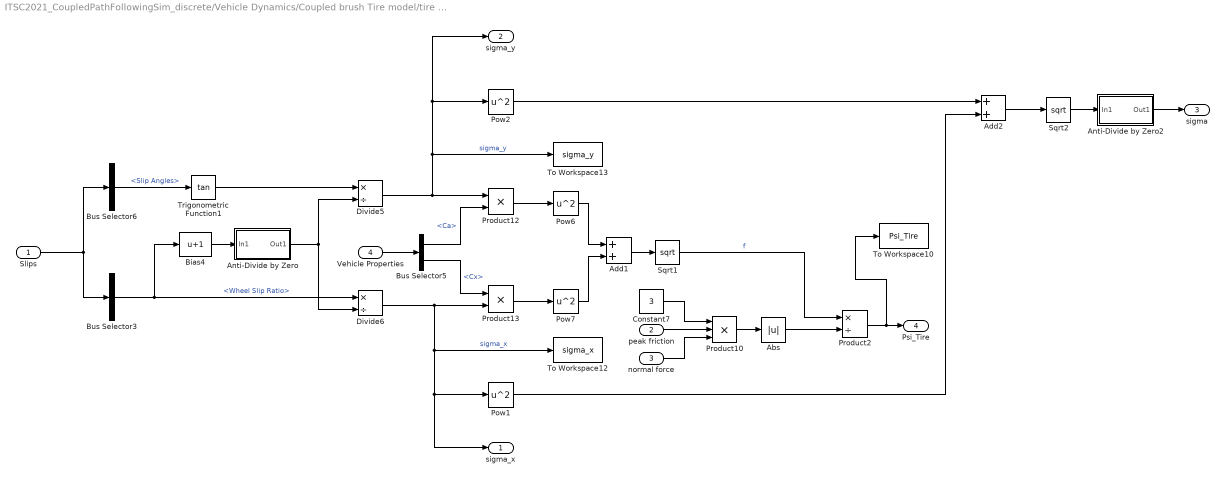
== system ITSC2021_CoupledPathFollowingSim_discrete/Vehicle Dynamics/Coupled brush Tire model/tire slip ==
  Slips : Inport
  peak friction : Inport  Port=2
  normal force : Inport  Port=3
  Vehicle Properties : Inport  Port=4
  Abs : Abs
  Add1 : Sum
  Add2 : Sum
  Anti-Divide by Zero : Subsystem
  Anti-Divide by Zero2 : Subsystem
  Bias4 : Bias  Bias=1
  Bus Selector3 : BusSelector  OutputSignals=Wheel Slip Ratio
  Bus Selector5 : BusSelector  OutputSignals=Ca,Cx
  Bus Selector6 : BusSelector  OutputSignals=Slip Angles
  Constant7 : Constant  Value=3
  Divide5 : Product  Inputs=*/
  Divide6 : Product  Inputs=*/
  Pow{1..2,6..7} (4 alike) : Math  Operator=square  SaturateOnIntegerOverflow=on
  Product10 : Product  Inputs=3  RndMeth=Zero
  Product12 : Product  RndMeth=Zero
  Product13 : Product  RndMeth=Zero
  Product2 : Product  Inputs=*/  RndMeth=Zero
  Sqrt1 : Sqrt  SaturateOnIntegerOverflow=on
  Sqrt2 : Sqrt  SaturateOnIntegerOverflow=on
  To Workspace10 : ToWorkspace  VariableName=Psi_Tire  SampleTime=-1
  To Workspace12 : ToWorkspace  VariableName=sigma_x  SampleTime=-1
  To Workspace13 : ToWorkspace  VariableName=sigma_y  SampleTime=-1
  Trigonometric Function1 : Trigonometry  Operator=tan
  sigma_x : Outport
  sigma_y : Outport  Port=2
  sigma : Outport  Port=3
  Psi_Tire : Outport  Port=4
  wires:
  Sqrt2/1 -> Anti-Divide by Zero2/1(In1)
  Pow7/1 -> Add1/2
  Slips/1 -> Bus Selector6/1, Bus Selector3/1
  normal force/1 -> Product10/3
  Product12/1 -> Pow6/1
  Sqrt1/1 -> Product2/1  "f"
  Bus Selector5/2 -> Product13/1  "<Cx>"
  Pow2/1 -> Add2/1
  peak friction/1 -> Product10/2
  Product10/1 -> Abs/1
  Anti-Divide by Zero/1(Out1) -> Divide6/2, Divide5/2
  Constant7/1 -> Product10/1
  Pow1/1 -> Add2/2
  Trigonometric Function1/1 -> Divide5/1
  Add2/1 -> Sqrt2/1
  Divide6/1 -> To Workspace12/1, sigma_x/1, Pow1/1, Product13/2  "sigma_x"
  Product13/1 -> Pow7/1
  Bus Selector3/1 -> Divide6/1, Bias4/1  "<Wheel Slip Ratio>"
  Pow6/1 -> Add1/1
  Divide5/1 -> To Workspace13/1, sigma_y/1, Pow2/1, Product12/1  "sigma_y"
  Product2/1 -> To Workspace10/1, Psi_Tire/1
  Vehicle Properties/1 -> Bus Selector5/1
  Bus Selector6/1 -> Trigonometric Function1/1  "<Slip Angles>"
  Bias4/1 -> Anti-Divide by Zero/1(In1)
  Bus Selector5/1 -> Product12/2  "<Ca>"
  Add1/1 -> Sqrt1/1
  Abs/1 -> Product2/2
  Anti-Divide by Zero2/1(Out1) -> sigma/1

== system ITSC2021_CoupledPathFollowingSim_discrete/Vehicle Dynamics/Vehicle Newtonian Dynamics/4 Wheel ax ==
  Bank Angle : Inport
  Road Grade : Inport  Port=2
  "Fx " : Inport  Port=3
  Add2 : Sum  Inputs=-+
  Bus Selector6 : BusSelector  OutputSignals=m
  Bus Selector7 : BusSelector  OutputSignals=m
  Divide2 : Product  Inputs=/*
  G : Constant  Value=9.81
  Product10 : Product  Inputs=4  RndMeth=Zero
  Sum of Elements3 : Sum  Inputs=+
  sin11 : Trigonometry  Operator=cos
  sin12 : Trigonometry
  ax : Outport
  wires:
  [Vehicle] -> Bus Selector6/1
  [Vehicle] -> Bus Selector7/1
  Add2/1 -> Divide2/2
  Bus Selector7/1 -> Divide2/1  "<m>"
  Divide2/1 -> ax/1
  Product10/1 -> Add2/1
  Sum of Elements3/1 -> Add2/2
  Bus Selector6/1 -> Product10/3  "<m>"
  G/1 -> Product10/4
  sin12/1 -> Product10/2
  sin11/1 -> Product10/1
  Bank Angle/1 -> sin11/1
  Road Grade/1 -> sin12/1
  "Fx "/1 -> Sum of Elements3/1

== system ITSC2021_CoupledPathFollowingSim_discrete/Vehicle Dynamics/Vehicle Newtonian Dynamics/4 Wheel ay ==
  Fy : Inport
  Bank Angle : Inport  Port=2
  Add : Sum
  Bus Selector2 : BusSelector  OutputSignals=m
  Bus Selector5 : BusSelector  OutputSignals=m
  Divide1 : Product  Inputs=*/
  G : Constant  Value=9.81
  Product4 : Product  Inputs=3  RndMeth=Zero
  Sum of Elements : Sum  Inputs=+
  sin : Trigonometry
  ay : Outport
  wires:
  [Vehicle] -> Bus Selector2/1
  Fy/1 -> Sum of Elements/1
  Product4/1 -> Add/2
  Add/1 -> Divide1/1
  Bus Selector2/1 -> Divide1/2  "<m>"
  Divide1/1 -> ay/1
  [Vehicle] -> Bus Selector5/1
  G/1 -> Product4/1
  Bus Selector5/1 -> Product4/2  "<m>"
  sin/1 -> Product4/3
  Bank Angle/1 -> sin/1
  Sum of Elements/1 -> Add/1

== system ITSC2021_CoupledPathFollowingSim_discrete/Vehicle Dynamics/Vehicle Newtonian Dynamics/4 Wheel rdot ==
  Fy : Inport
  Fx : Inport  Port=2
  Add1 : Sum
  Add2 : Sum  Inputs=-++
  Add3 : Sum  Inputs=-+
  Add4 : Sum  Inputs=-+
  Bus Selector1 : BusSelector  OutputSignals=b
  Bus Selector2 : BusSelector  OutputSignals=a
  Bus Selector3 : BusSelector  OutputSignals=d
  Bus Selector7 : BusSelector  OutputSignals=Izz
  Demux : Demux
  Divide2 : Product  Inputs=/*
  Gain : Gain  Gain=1/2
  Product1 : Product  RndMeth=Zero
  Product2 : Product  RndMeth=Zero
  Product5 : Product  RndMeth=Zero
  Selector : Selector  InputPortWidth=4  IndexOptions=Index vector (dialog)  Indices=[3 4]  OutputSizes=1
  Selector1 : Selector  InputPortWidth=4  IndexOptions=Index vector (dialog)  Indices=[1 2]  OutputSizes=1
  Sum of Elements : Sum  Inputs=+
  Sum of Elements1 : Sum  Inputs=+
  rdot : Outport
  wires:
  Fy/1 -> Selector/1, Selector1/1
  Divide2/1 -> rdot/1
  Bus Selector7/1 -> Divide2/1  "<Izz>"
  Add2/1 -> Divide2/2
  [Vehicle] -> Bus Selector7/1
  [Vehicle] -> Bus Selector1/1
  Selector/1 -> Sum of Elements/1
  Selector1/1 -> Sum of Elements1/1
  Sum of Elements/1 -> Product1/1
  Bus Selector1/1 -> Product1/2  "<b>"
  Product1/1 -> Add2/1
  Fx/1 -> Demux/1
  [Vehicle] -> Bus Selector2/1
  Product2/1 -> Add2/2
  Bus Selector2/1 -> Product2/1  "<a>"
  Sum of Elements1/1 -> Product2/2
  Demux/3 -> Add3/1
  Demux/4 -> Add3/2
  Demux/1 -> Add4/1
  Demux/2 -> Add4/2
  Add4/1 -> Add1/1
  [Vehicle] -> Bus Selector3/1
  Add1/1 -> Product5/2
  Bus Selector3/1 -> Gain/1  "<d>"
  Gain/1 -> Product5/1
  Product5/1 -> Add2/3
  Add3/1 -> Add1/2

== system ITSC2021_CoupledPathFollowingSim_discrete/Vehicle Dynamics/Vehicle Newtonian Dynamics/Wheel to Body Transform ==
  Delta : Inport
  Fy_Wheel : Inport  Port=2
  Fx_Wheel : Inport  Port=3
  Add : Sum
  Cos1 : Trigonometry  Operator=cos
  Cos2 : Trigonometry
  Cos8 : Trigonometry  Operator=cos
  Cos9 : Trigonometry
  Fx_Wheel1 : InportShadow  Port=3
  Fy_Wheel1 : InportShadow  Port=2
  Product{4..7} (4 alike) : Product
  Subtract : Sum  Inputs=+-
  Fy_Body : Outport
  Fx_Body : Outport  Port=2
  wires:
  Subtract/1 -> Fx_Body/1
  Delta/1 -> Cos8/1, Cos9/1, Cos2/1, Cos1/1
  Cos8/1 -> Product4/1
  Cos9/1 -> Product5/1
  Cos1/1 -> Product6/1
  Cos2/1 -> Product7/1
  Fx_Wheel1/1 -> Product7/2
  Fy_Wheel1/1 -> Product6/2
  Fy_Wheel/1 -> Product5/2
  Fx_Wheel/1 -> Product4/2
  Product4/1 -> Subtract/1
  Product5/1 -> Subtract/2
  Product6/1 -> Add/1
  Product7/1 -> Add/2
  Add/1 -> Fy_Body/1

== system ITSC2021_CoupledPathFollowingSim_discrete/Subsystem1/Friction Estimator/fric est Calculate Normals/Normal Force Lateral Transfer ==
  Accelerations : Inport
  Bus Selector1 : BusSelector  OutputSignals=a_y_out
  Bus Selector4 : BusSelector  OutputSignals=b,L,a
  Bus Selector6 : BusSelector  OutputSignals=m,h_cg,d
  Delay1 : Delay  DelayLength=1  InitialCondition=0
  Divide3 : Product  Inputs=*/
  Divide4 : Product  Inputs=/*
  Gain2 : Gain  Gain=0
  Product{1..2,4..5} (4 alike) : Product  RndMeth=Zero
  Product3 : Product  Inputs=*/  RndMeth=Zero
  Lateral Transfer Front : Outport
  Lateral Transfer Rear : Outport  Port=2
  wires:
  Divide3/1 -> Product2/2
  Bus Selector4/2 -> Divide3/2, Divide4/1  "<L>"
  Bus Selector4/1 -> Divide3/1  "<b>"
  Gain2/1 -> Product5/1
  Product2/1 -> Lateral Transfer Front/1
  Product5/1 -> Product2/1, Product1/2
  Bus Selector6/2 -> Product3/1  "<h_cg>"
  Product1/1 -> Lateral Transfer Rear/1
  Bus Selector6/1 -> Product4/2  "<m>"
  Accelerations/1 -> Delay1/1
  Delay1/1 -> Bus Selector1/1
  Divide4/1 -> Product1/1
  Bus Selector1/1 -> Product4/1  "<a_y_out>"
  Bus Selector6/3 -> Product3/2  "<d>"
  [Vehicle] -> Bus Selector4/1
  [Vehicle] -> Bus Selector6/1
  Bus Selector4/3 -> Divide4/2  "<a>"
  Product4/1 -> Gain2/1
  Product3/1 -> Product5/2

== system ITSC2021_CoupledPathFollowingSim_discrete/Subsystem1/Friction Estimator/fric est Calculate Normals/Normal Force Longitudinal Transfer ==
  Accelerations : Inport
  Bus Selector2 : BusSelector  OutputSignals=m,L,h_cg
  Bus Selector3 : BusSelector  OutputSignals=a_x_out
  Delay : Delay  DelayLength=1  InitialCondition=0
  Divide1 : Product  Inputs=/*
  Gain1 : Gain  Gain=0
  Gain3 : Gain  Gain=2
  Product1 : Product  RndMeth=Zero
  Product2 : Product  RndMeth=Zero
  Half Long Transfer : Outport
  wires:
  Bus Selector2/2 -> Gain3/1  "<L>"
  Gain1/1 -> Product1/1
  Bus Selector2/3 -> Divide1/2  "<h_cg>"
  Divide1/1 -> Product1/2
  [Vehicle] -> Bus Selector2/1
  Accelerations/1 -> Delay/1
  Bus Selector2/1 -> Product2/2  "<m>"
  Bus Selector3/1 -> Product2/1  "<a_x_out>"
  Product2/1 -> Gain1/1
  Product1/1 -> Half Long Transfer/1
  Gain3/1 -> Divide1/1
  Delay/1 -> Bus Selector3/1

== system ITSC2021_CoupledPathFollowingSim_discrete/Subsystem1/Friction Estimator/fric est Calculate Normals/Normal Force Static ==
  Road Geometry : Inport
  " " : Product  RndMeth=Zero
  Add : Sum
  Bus Selector : BusSelector  OutputSignals=Grade
  Bus Selector1 : BusSelector  OutputSignals=m,L,h_cg,b,a
  Bus Selector2 : BusSelector  OutputSignals=Grade
  Divide : Product  Inputs=*/
  Gain : Gain  Gain=2
  Product1 : Product  RndMeth=Zero
  Product3 : Product  Inputs=3  RndMeth=Zero
  Product4 : Product  RndMeth=Zero
  Road Geometry1 : InportShadow
  Subtract : Sum  Inputs=-+
  Trigonometric Function : Trigonometry  Operator=cos
  Trigonometric Function1 : Trigonometry  Operator=tan
  g : Constant  Value=9.81
  Half Static Front : Outport
  Half Static Rear : Outport  Port=2
  wires:
  Product4/1 -> Add/1, Subtract/1
  Add/1 -> Product1/2
  g/1 -> Product3/2
  [Vehicle] -> Bus Selector1/1
  Bus Selector1/4 -> Subtract/2  "<b>"
  Product3/1 -> Divide/1
  Bus Selector1/1 -> Product3/3  "<m>"
  Trigonometric Function/1 -> Product3/1
  Bus Selector1/5 -> Add/2  "<a>"
  Bus Selector1/3 -> Product4/2  "<h_cg>"
  Trigonometric Function1/1 -> Product4/1
  Divide/1 -> Product1/1, " "/1
  Bus Selector/1 -> Trigonometric Function/1  "<Grade>"
  Bus Selector1/2 -> Gain/1  "<L>"
  Subtract/1 -> " "/2
  Gain/1 -> Divide/2
  Road Geometry/1 -> Bus Selector/1
  Product1/1 -> Half Static Rear/1
  " "/1 -> Half Static Front/1
  Road Geometry1/1 -> Bus Selector2/1
  Bus Selector2/1 -> Trigonometric Function1/1  "<Grade>"

== system ITSC2021_CoupledPathFollowingSim_discrete/Vehicle Dynamics/Calculate Slips/Wheel Slip Ratio this block is wrong because it use vehicle body velocity to calculate slip ratio/Anti-Divide by Zero ==
  In1 : Inport
  Add : Sum
  Compare To Zero : simulink/Logic and Bit Operations/Compare To Zero  relop===  OutDataTypeStr=boolean
  Constant : Constant  Value=eps
  Product : Product
  Out1 : Outport
  wires:
  In1/1 -> Add/1, Compare To Zero/1
  Product/1 -> Add/2
  Constant/1 -> Product/2
  Compare To Zero/1 -> Product/1
  Add/1 -> Out1/1

== system ITSC2021_CoupledPathFollowingSim_discrete/Vehicle Dynamics/Calculate Slips/Wheel Slip Ratio1/Anti-Divide by Zero ==
  In1 : Inport
  Add : Sum
  Compare To Zero : simulink/Logic and Bit Operations/Compare To Zero  relop===  OutDataTypeStr=boolean
  Constant : Constant  Value=eps
  Product : Product
  Out1 : Outport
  wires:
  In1/1 -> Add/1, Compare To Zero/1
  Product/1 -> Add/2
  Constant/1 -> Product/2
  Compare To Zero/1 -> Product/1
  Add/1 -> Out1/1

== system ITSC2021_CoupledPathFollowingSim_discrete/Vehicle Dynamics/Coupled brush Tire model/Wheel Forces/Anti-Divide by Zero ==
  In1 : Inport
  Add : Sum
  Compare To Zero : simulink/Logic and Bit Operations/Compare To Zero  relop===  OutDataTypeStr=boolean
  Constant : Constant
  Product : Product
  Out1 : Outport
  wires:
  Add/1 -> Out1/1
  Compare To Zero/1 -> Product/1
  Constant/1 -> Product/2
  Product/1 -> Add/2
  In1/1 -> Compare To Zero/1, Add/1

== system ITSC2021_CoupledPathFollowingSim_discrete/Vehicle Dynamics/Coupled brush Tire model/tire slip/Anti-Divide by Zero ==
  In1 : Inport
  Add : Sum
  Compare To Zero : simulink/Logic and Bit Operations/Compare To Zero  relop===  OutDataTypeStr=boolean
  Constant : Constant  Value=eps
  Product : Product
  Out1 : Outport
  wires:
  Add/1 -> Out1/1
  Compare To Zero/1 -> Product/1
  Constant/1 -> Product/2
  Product/1 -> Add/2
  In1/1 -> Compare To Zero/1, Add/1

== system ITSC2021_CoupledPathFollowingSim_discrete/Vehicle Dynamics/Coupled brush Tire model/tire slip/Anti-Divide by Zero2 ==
  In1 : Inport
  Add : Sum
  Compare To Zero : simulink/Logic and Bit Operations/Compare To Zero  relop===  OutDataTypeStr=boolean
  Constant : Constant  Value=eps
  Product : Product
  Out1 : Outport
  wires:
  Add/1 -> Out1/1
  Compare To Zero/1 -> Product/1
  Constant/1 -> Product/2
  Product/1 -> Add/2
  In1/1 -> Compare To Zero/1, Add/1

== matlab function ITSC2021_CoupledPathFollowingSim_discrete/Subsystem1/Noise Models/GPS Noise Function ==
  settings: updateMethod=DISCRETE
  data: v_x input; v_x_out output; v_y input; r input; sampling_time input; v_y_out output; r_out output
function [v_x_out, v_y_out, r_out] = GPS_noise(v_x, v_y, r, sampling_time)

% v_x: velocity in X direction [m/s]
% v_y: velocity in Y direction [m/s]
% r: the yaw rate [rad/s]
% sample_rate: frequency at which velocities are being calculated [Hz]

% sensor specifications
sigma_x = 0.025;
sigma_y = 0.025;
sigma_theta = 0.009;

% simulate noisy measurements
v_x_out = v_x + normrnd(0,1.4142*sigma_x)*sampling_time;
v_y_out = v_y + normrnd(0,1.4142*sigma_y)*sampling_time;
r_out   = r + normrnd(0,1.4142*sigma_theta)*sampling_time;

end

== matlab function ITSC2021_CoupledPathFollowingSim_discrete/Vehicle Controller/Driver Model/Drive Line/MATLAB Function ==
  settings: updateMethod=DISCRETE
  data: measured_speed input; command_speed input; torque output; error_D output; error_I output
% Purpose: PID controller block. Tune the values of Kp,Ki,Kd to obtain
% desired contol performance 
% input: desired speed and measured feedback speed
% ouput: contol voltage. integral and derivative of error 

function [torque,error_D, error_I] = PID_controller(measured_speed,command_speed)

% Initialization
%A persistent variable is a local variable in a MATLAB function that retains 
% its value in memory between calls to the function. 
% For code generation, functions must initialize a persistent variable if it is empty. 

persistent flag;
persistent error_integral;
persistent mid;
persistent delta_t;
persistent error;
persistent Kp; %Proportional gain
persistent Ki; %Integral gain
persistent Kd; % Differentiation gain
persistent Kff; % Velocity feed-forward gain
persistent Kaw; % Anti-windup gain ,refer to https://www.mathworks.com/help/autoblks/ref/longitudinaldriver.html
persistent counts;
if isempty(flag)
    flag = 1;
    error_integral= 0;
    mid = 0;
    delta_t = 0.01; %100Hz
    error = 0;

    Kd = 0;
    counts =1;
end

counts= counts +1;
%control error  
error = command_speed - measured_speed;

if error>0.1 %need to speed up
    
    Kp = 200;
    Ki = 0;
elseif error<=0.1 && error> -0.1 
    Kp = 200;
    Ki = 0;
elseif error<= -0.1 %&& counts<2000
    Kp = 660;
    Ki = 0; %
else
    Kp = 200;
    Ki = 0; %-20
end
% derivative 
error_last= mid;
mid = error;
error_D = (error -error_last)/delta_t;

% integral
error_integral = error_integral + error*delta_t;
error_I = error_integral;


% if mod(counts,100)==0
%     counts =0;
%     error_I= 0;
% end
% if counts  == 2000
%     error_I = 0;
% end

% PID contoller output
torque = Kp*error  + Ki* error_I + Kd*error_D ;

== matlab function ITSC2021_CoupledPathFollowingSim_discrete/Subsystem1/Noise Models/IMU Noise Function ==
  settings: updateMethod=DISCRETE
  data: a_x input; a_x_out output; a_y input; sampling_time input; a_y_out output
function [a_x_out, a_y_out] = IMU_noise(a_x, a_y, sampling_time)

% a_x: accelaration in X direction [m/s^2]
% a_y: accelaration in Y direction [m/s^2]
% alpha: the yaw angular accelaration [rad/s^2]
% sample_rate: frequency at which velocities are being calculated [Hz]

% sensor specifications
sigma_x = 0.25;
sigma_y = 0.25;
% sigma_theta = 0.09;

% simulate noisy measurements
a_x_out = a_x + normrnd(0,2*sigma_x)*(sampling_time^2);
a_y_out = a_y + normrnd(0,2*sigma_y)*(sampling_time^2);
% alpha_out = alpha_in + normrnd(0,2*sigma_theta)*(sampling_time^2);

end

== matlab function ITSC2021_CoupledPathFollowingSim_discrete/Subsystem/ST Friction DB Query/MATLAB Function ==
  data: y output; time input
% Purpose: calculate some friction data
% input: time
%
% ouput: friction data of 4 wheels

function y = fric_generator(time)

% Initialization
%A persistent variable is a local variable in a MATLAB function that retains
% its value in memory between calls to the function.
% For code generation, functions must initialize a persistent variable if it is empty.
if time< 150
    y = 0.9*ones(4,1);
elseif time>= 150 && time< 250
    y = 0.8*ones(4,1);
elseif time>= 250 && time< 500
    y = 0.95*ones(4,1);
elseif time>= 500 && time< 600
    y = 0.75*ones(4,1);
elseif time>= 600 && time< 750
    y = 0.9*ones(4,1);

else
    y = (0.85+0.15*sin(time*2*pi/200))*ones(4,1);
    
end

== matlab function ITSC2021_CoupledPathFollowingSim_discrete/Subsystem/ST Friction DB Query/MATLAB Function wheel Position ==
  settings: updateMethod=DISCRETE
  data: P_FL output; P_FR output; P_RL output; P_CG input; P_RR output; Veh_Geo input
% Purpose: calculate the 4 wheels geographical ENU postion 
% input: current vehicle CG location, array(E,N,U,heading),meters, degree
%        Veh_Geo,array(a, b, T, h), units: meter
% ouput: location of 4 wheels
%        P_FL, array(E,N,U),meter
%
%
%
% Assumption: 2D plane, i.e. ignore up temporarily
%             azimuth:The reference plane for an azimuth is typically true north,
%                     measured as a 0° azimuth. Moving clockwise on a 360 degree
%                     circle, east has azimuth 90°, south 180°, and west 270
%             yaw, the same with azimuth

function [P_FL,P_FR,P_RL,P_RR] = wheel_postion(P_CG,Veh_Geo)

% Initialization
%A persistent variable is a local variable in a MATLAB function that retains 
% its value in memory between calls to the function. 
% For code generation, functions must initialize a persistent variable if it is empty. 
persistent flag;
persistent len_FL;
persistent len_FR;
persistent len_RL;
persistent len_RR;
persistent az_FL;
persistent az_FR;
persistent az_RL;
persistent az_RR;
persistent yaw;

if isempty(flag)
    flag = 1;
    len_FL = 0; %distance from CG to front left wheel
    len_FR = 0; %distance from CG to front right wheel
    len_RL = 0; %distance from CG to rear left wheel
    len_RR = 0; %distance from CG to rear right wheel
    
    az_FL = 0; %azimuth of front left wheel, 
    az_FR = 0;
    az_RL = 0;
    az_RR = 0;
    yaw = P_CG(4)*180/pi; %degree
    
end
yaw = 90-P_CG(4)*180/pi; %degree

if yaw < 0 
    yaw = 360+ yaw;
end
% position of front left wheel
len_FL = hypot(Veh_Geo(1),Veh_Geo(3)/2); % meters
az_FL = yaw - atan2d(Veh_Geo(3)/2,Veh_Geo(1)); % degree
P_FL = [P_CG(1)+len_FL*sind(az_FL); P_CG(2)+len_FL*cosd(az_FL); P_CG(3)];
%P_FL = [P_CG(1)+0*len_FL*sind(az_FL) P_CG(2)+0*len_FL*cosd(az_FL) P_CG(3)];

% position of front right wheel
len_FR = len_FL;
az_FR = yaw+ atan2d(Veh_Geo(3)/2,Veh_Geo(1)); % degree
P_FR = [P_CG(1)+len_FR*sind(az_FR); P_CG(2)+len_FR*cosd(az_FR); P_CG(3)];

% position of rear left wheel
len_RL = hypot(Veh_Geo(2),Veh_Geo(3)/2);
az_RL = yaw + 180 + atan2d(Veh_Geo(3)/2,Veh_Geo(2));
P_RL = [P_CG(1)+len_RL*sind(az_RL) ;P_CG(2)+len_RL*cosd(az_RL); P_CG(3)];

% position of rear right wheel
len_RR = len_RL;
az_RR = yaw+ 180 - atan2d(Veh_Geo(3)/2,Veh_Geo(2));
P_RR = [P_CG(1)+len_RR*sind(az_RR); P_CG(2)+len_RR*cosd(az_RR); P_CG(3)];
